simulink model "sampleModel1702_4_sub_sub_sub"  (R2023a)
settings: Solver=VariableStepAuto  StartTime=0.0  StopTime=10.0  RelTol=1e-3
libraries: hdlsllib x4, simulink x2
settings Model: Creator=user1  LastModifiedBy=user1
settings OptimizationCC: BlockReduction=off  ConditionallyExecuteInputs=off

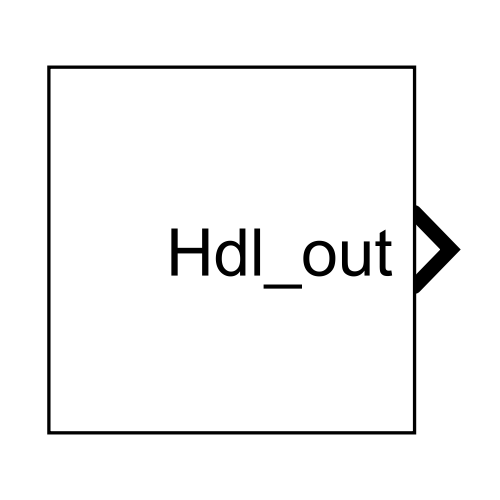
[thumbnail: Simulink's stored preview of the top-level diagram]
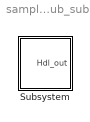
== system sampleModel1702_4_sub_sub_sub ==
  Subsystem : Subsystem

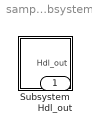
== system sampleModel1702_4_sub_sub_sub/Subsystem ==
  Subsystem : Subsystem
  Hdl_out : Outport  OutDataTypeStr=uint8

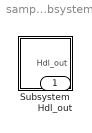
== system sampleModel1702_4_sub_sub_sub/Subsystem/Subsystem ==
  Subsystem : Subsystem
  Hdl_out : Outport  OutDataTypeStr=uint8

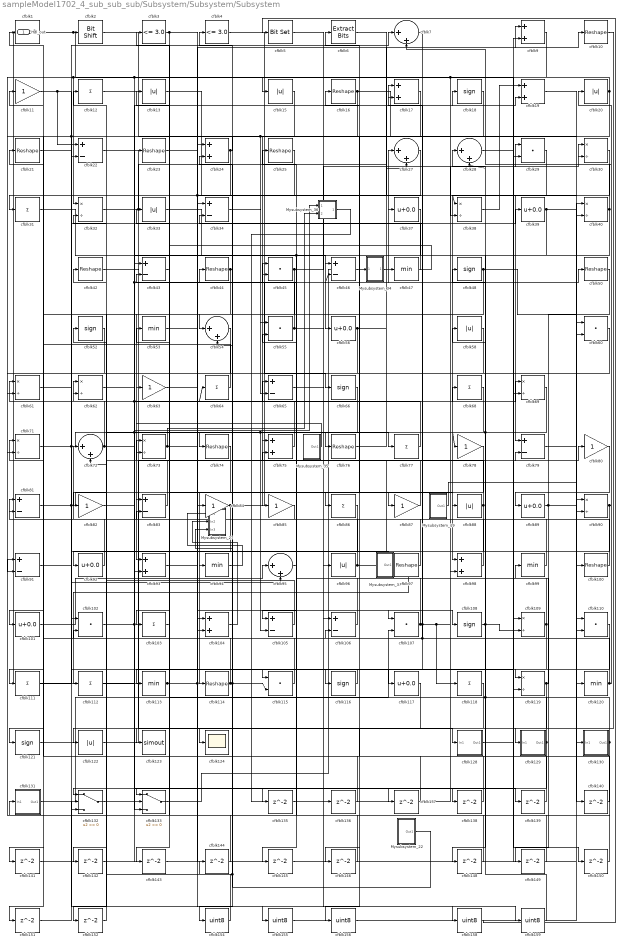
== system sampleModel1702_4_sub_sub_sub/Subsystem/Subsystem/Subsystem ==
  Mysubsystem_19 : Subsystem  TreatAsAtomicUnit=on  RTWFcnName=Mysubsystem_19
      settings: RTWFcnNameOpts=User specified  RTWFileNameOpts=Use function name
  Mysubsystem_22 : Subsystem  TreatAsAtomicUnit=on  RTWFcnName=Mysubsystem_22
      settings: RTWFcnNameOpts=User specified  RTWFileNameOpts=Use function name
  Mysubsystem_27 : Subsystem  TreatAsAtomicUnit=on  RTWFcnName=Mysubsystem_27
      settings: RTWFcnNameOpts=User specified  RTWFileNameOpts=Use function name
  Mysubsystem_34 : Subsystem  TreatAsAtomicUnit=on  RTWFcnName=Mysubsystem_34
      settings: RTWFcnNameOpts=User specified  RTWFileNameOpts=Use function name
  Mysubsystem_35 : Subsystem  TreatAsAtomicUnit=on  RTWFcnName=Mysubsystem_35
      settings: RTWFcnNameOpts=User specified  RTWFileNameOpts=Use function name
  Mysubsystem_36 : Subsystem  TreatAsAtomicUnit=on  RTWFcnName=Mysubsystem_36
      settings: RTWFcnNameOpts=User specified  RTWFileNameOpts=Use function name
  Mysubsystem_37 : Subsystem  TreatAsAtomicUnit=on  RTWFcnName=Mysubsystem_37
      settings: RTWFcnNameOpts=User specified  RTWFileNameOpts=Use function name
  cfblk1 : ArithShift  BitShiftNumber=8
  cfblk{10,16,21,23,25,42,44,50,74,76,97,100,114} (13 alike) : Reshape
  cfblk{37,39,56,89,92,101,117} (7 alike) : Bias  Bias=0.0  SaturateOnIntegerOverflow=off
  cfblk{29,45,55,60,102,107,110,115} (8 alike) : DotProduct  OutDataTypeStr=uint8
  cfblk{12,31,64,68,77,86,103,111..112,118} (10 alike) : Sum  Inputs=+  OutDataTypeStr=uint8
  cfblk{9,17,19,24,75,93,98,104} (8 alike) : Sum  OutDataTypeStr=uint8
  cfblk{22,34,43,46,65,79,81,83,91,105..106} (11 alike) : Sum  Inputs=+-  OutDataTypeStr=uint8
  cfblk{18,48,52,66,108,116,121} (7 alike) : Signum
  cfblk{30,32,38,40,61..62,69,71,73,90,109,119} (12 alike) : Product  Inputs=*/  OutDataTypeStr=uint8  RndMeth=Zero  SaturateOnIntegerOverflow=on
  cfblk{11,63,78,80,82,84..85,87} (8 alike) : Gain  OutDataTypeStr=uint8
  cfblk{47,53,94,99,113,120} (6 alike) : MinMax  OutDataTypeStr=uint8
  cfblk{13,15,20,33,58,88,96,122} (8 alike) : Abs  OutDataTypeStr=uint8  SaturateOnIntegerOverflow=off
  cfblk123 : ToWorkspace  VariableName=simout  SaveFormat=Timeseries  SampleTime=-1
  cfblk124 : Scope
  cfblk128 : Subsystem
      settings: LibrarySourceBlock=|
      | hdlsllib/Ports &
      | Subsystems/Subsystem
  cfblk129 : Subsystem
      settings: LibrarySourceBlock=|
      | hdlsllib/Ports &
      | Subsystems/Subsystem
  cfblk130 : Subsystem
      settings: LibrarySourceBlock=|
      | hdlsllib/Ports &
      | Subsystems/Subsystem
  cfblk131 : Subsystem
      settings: LibrarySourceBlock=|
      | hdlsllib/Ports &
      | Subsystems/Subsystem
  cfblk132 : Switch  OutDataTypeStr=uint8  SaturateOnIntegerOverflow=off  InputSameDT=off
  cfblk133 : Switch  OutDataTypeStr=uint8  SaturateOnIntegerOverflow=off  InputSameDT=off
  cfblk{135..146,148..152} (17 alike) : Delay  SampleTime=1
  cfblk{154..156,158..159} (5 alike) : DataTypeConversion  OutDataTypeStr=uint8  SaturateOnIntegerOverflow=off  RndMeth=Floor
  cfblk2 : hdlsllib/Logic and Bit Operations/Bit Shift  mode=Shift Left Logical  N=0
  cfblk{7,27..28,54,72,95} (6 alike) : Sum  Inputs=|++  OutDataTypeStr=uint8
  cfblk3 : hdlsllib/Logic and Bit Operations/Compare To Constant  relop=<=  const=3.0  OutDataTypeStr=uint8
  cfblk4 : hdlsllib/Logic and Bit Operations/Compare To Constant  relop=<=  const=3.0  OutDataTypeStr=uint8
  cfblk5 : simulink/Logic and Bit Operations/Bit Set  iBit=0
      settings: LibrarySourceBlock=|
      | hdlsllib/Logic and Bit
      | Operations/Bit Set
  cfblk6 : simulink/Logic and Bit Operations/Extract Bits  bitsToExtract=Upper half  numBits=8  bitIdxRange=[0 7]  outScalingMode=Preserve fixed-point scaling
      settings: LibrarySourceBlock=|
      | hdlsllib/Logic and Bit
      | Operations/Extract Bits
  Hdl_out : Outport  OutDataTypeStr=uint8
  wires:
  cfblk122/1 -> cfblk80/1
  cfblk80/1 -> cfblk89/1
  cfblk9/1 -> cfblk38/2, cfblk71/2, cfblk32/1
  cfblk113/1 -> Hdl_out/1, cfblk137/1, cfblk69/1
  cfblk42/1 -> cfblk128/1(In1)
  cfblk72/1 -> cfblk62/1, Mysubsystem_36/1(In1)
  cfblk44/1 -> cfblk54/2, cfblk93/1
  cfblk31/1 -> cfblk56/1
  cfblk88/1 -> cfblk122/1, cfblk16/1
  cfblk105/1 -> cfblk12/1
  cfblk56/1 -> cfblk141/1, cfblk27/2
  cfblk120/1 -> cfblk20/1, cfblk17/1, cfblk71/1
  cfblk10/1 -> cfblk129/1(In1)
  cfblk84/1 -> cfblk104/2, cfblk50/1
  cfblk66/1 -> cfblk74/1
  cfblk71/1 -> cfblk119/2, cfblk77/1
  cfblk22/1 -> cfblk114/1
  cfblk27/1 -> cfblk85/1
  cfblk38/1 -> cfblk19/1
  cfblk30/1 -> cfblk98/1
  cfblk17/1 -> cfblk75/1
  cfblk18/1 -> cfblk86/1
  cfblk81/1 -> cfblk39/1, cfblk88/1
  cfblk74/1 -> cfblk103/1
  cfblk132/1 -> cfblk23/1
  cfblk46/1 -> cfblk27/1
  cfblk25/1 -> cfblk31/1
  cfblk13/1 -> cfblk100/1
  cfblk77/1 -> cfblk61/1
  cfblk48/1 -> cfblk151/1, cfblk60/2
  cfblk4/1 -> cfblk66/1
  cfblk24/1 -> cfblk4/1, cfblk101/1
  cfblk83/1 -> cfblk62/2
  cfblk60/1 -> cfblk92/1
  cfblk39/1 -> cfblk133/3, cfblk130/1(In1)
  cfblk52/1 -> cfblk121/1
  cfblk90/1 -> cfblk105/1, cfblk30/1
  cfblk76/1 -> cfblk19/2
  cfblk85/1 -> cfblk83/2
  cfblk54/1 -> cfblk61/2
  cfblk95/1 -> cfblk45/1
  cfblk16/1 -> cfblk91/2, cfblk90/1
  cfblk115/1 -> cfblk73/1
  cfblk101/1 -> cfblk95/1
  cfblk102/1 -> cfblk139/1, cfblk17/2, cfblk64/1
  cfblk106/1 -> cfblk44/1
  cfblk15/1 -> cfblk124/1
  cfblk33/1 -> cfblk46/1
  cfblk111/1 -> cfblk7/1
  cfblk20/1 -> cfblk15/1, cfblk65/2, cfblk111/1, cfblk22/2
  cfblk103/1 -> cfblk53/1
  cfblk23/1 -> cfblk9/1
  cfblk91/1 -> cfblk102/1
  cfblk43/1 -> cfblk63/1
  cfblk78/1 -> cfblk94/1
  cfblk87/1 -> cfblk73/2
  cfblk3/1 -> cfblk133/1, cfblk155/1, cfblk38/1
  cfblk92/1 -> cfblk81/1
  cfblk2/1 -> cfblk96/1
  cfblk29/1 -> cfblk79/1
  cfblk12/1 -> cfblk109/1
  cfblk93/1 -> cfblk68/1
  cfblk45/1 -> cfblk82/1, cfblk30/2
  cfblk108/1 -> cfblk28/2, cfblk109/2
  cfblk32/1 -> cfblk104/1, cfblk10/1
  cfblk65/1 -> cfblk107/1
  cfblk63/1 -> cfblk47/1
  cfblk99/1 -> cfblk11/1
  cfblk1/1 -> cfblk2/1, cfblk69/2, cfblk43/1
  cfblk40/1 -> cfblk7/2, cfblk148/1, cfblk78/1
  cfblk64/1 -> cfblk21/1
  cfblk34/1 -> cfblk55/1
  cfblk96/1 -> cfblk79/2, cfblk42/1
  cfblk121/1 -> cfblk107/2
  cfblk37/1 -> cfblk145/1, cfblk54/1
  cfblk61/1 -> cfblk97/1
  cfblk11/1 -> cfblk22/1, cfblk95/2
  cfblk116/1 -> cfblk113/1
  cfblk98/1 -> cfblk72/1
  cfblk19/1 -> cfblk90/2
  cfblk86/1 -> cfblk115/1
  cfblk112/1 -> cfblk46/2, cfblk18/1
  cfblk55/1 -> cfblk13/1, cfblk106/1
  cfblk47/1 -> cfblk34/2
  cfblk89/1 -> cfblk149/1, cfblk40/1
  cfblk100/1 -> cfblk28/1
  cfblk131/1(Out1) -> cfblk84/1
  cfblk82/1 -> cfblk116/1
  cfblk53/1 -> cfblk108/1
  cfblk7/1 -> cfblk117/1
  cfblk68/1 -> cfblk105/2, cfblk133/2, cfblk132/1
  cfblk58/1 -> cfblk87/1
  cfblk130/1(Out1) -> cfblk6/1, cfblk131/1(In1)
  cfblk75/1 -> cfblk65/1
  cfblk119/1 -> cfblk156/1, cfblk99/1
  cfblk109/1 -> cfblk45/2, cfblk123/1
  cfblk97/1 -> cfblk3/1
  cfblk114/1 -> cfblk52/1, cfblk24/2, cfblk115/2
  cfblk107/1 -> cfblk25/1, cfblk37/1, cfblk118/1, cfblk29/1
  cfblk129/1(Out1) -> cfblk152/1, cfblk33/1, cfblk48/1
  cfblk128/1(Out1) -> cfblk29/2
  cfblk6/1 -> cfblk40/2
  cfblk73/1 -> cfblk76/1, Mysubsystem_36/2(In2)
  cfblk50/1 -> cfblk119/1
  cfblk62/1 -> cfblk135/1
  cfblk135/1 -> cfblk98/2
  cfblk136/1 -> cfblk72/2
  cfblk137/1 -> cfblk1/1
  cfblk69/1 -> cfblk138/1
  cfblk138/1 -> cfblk81/2
  cfblk139/1 -> cfblk106/2
  cfblk79/1 -> cfblk140/1
  cfblk140/1 -> cfblk75/2
  cfblk141/1 -> cfblk60/1
  cfblk118/1 -> cfblk142/1
  cfblk142/1 -> cfblk93/2
  cfblk143/1 -> cfblk34/1
  cfblk144/1 -> cfblk91/1
  cfblk145/1 -> cfblk9/2
  cfblk117/1 -> cfblk146/1
  cfblk146/1 -> cfblk55/2
  cfblk148/1 -> cfblk43/2
  cfblk149/1 -> cfblk132/2
  cfblk28/1 -> cfblk150/1
  cfblk150/1 -> cfblk24/1
  cfblk151/1 -> cfblk132/3
  cfblk152/1 -> cfblk32/2
  cfblk110/1 -> cfblk154/1
  cfblk154/1 -> cfblk144/1
  cfblk155/1 -> cfblk110/1
  cfblk156/1 -> cfblk110/2
  cfblk21/1 -> cfblk158/1
  cfblk158/1 -> cfblk5/1
  cfblk5/1 -> cfblk159/1
  cfblk159/1 -> cfblk58/1
  Mysubsystem_19/1(Out1) -> cfblk120/1
  Mysubsystem_22/1(Out1) -> cfblk102/2, Mysubsystem_27/3(In3)
  cfblk94/1 -> Mysubsystem_27/1(In1)
  cfblk104/1 -> Mysubsystem_27/2(In2)
  cfblk133/1 -> Mysubsystem_34/1(In1)
  Mysubsystem_34/1(Out1) -> cfblk143/1
  Mysubsystem_35/1(Out1) -> cfblk83/1
  Mysubsystem_36/1(Out1) -> cfblk136/1
  Mysubsystem_37/1(Out1) -> cfblk112/1

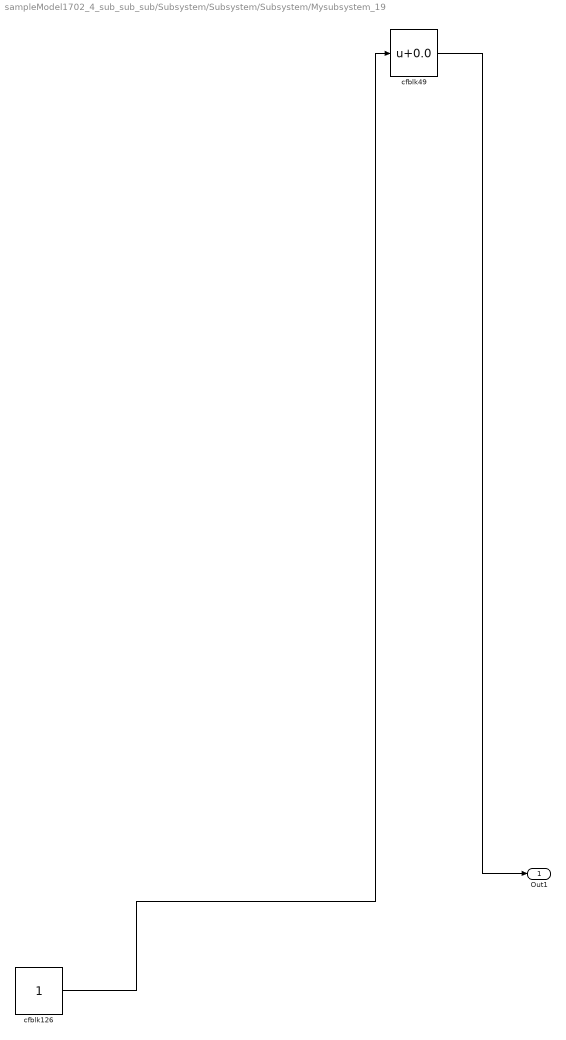
== system sampleModel1702_4_sub_sub_sub/Subsystem/Subsystem/Subsystem/Mysubsystem_19 ==
  cfblk126 : Constant  SampleTime=-1
  cfblk49 : Bias  Bias=0.0  SaturateOnIntegerOverflow=off
  Out1 : Outport
  wires:
  cfblk49/1 -> Out1/1
  cfblk126/1 -> cfblk49/1

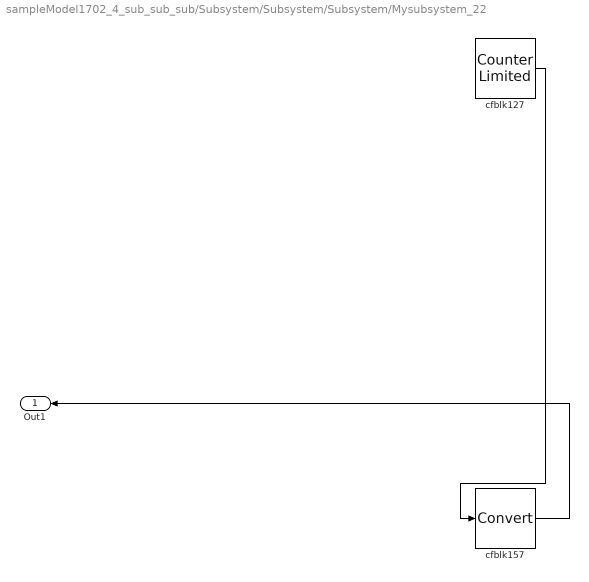
== system sampleModel1702_4_sub_sub_sub/Subsystem/Subsystem/Subsystem/Mysubsystem_22 ==
  cfblk127 : hdlsllib/Sources/Counter Limited  uplimit=7  tsamp=-1
  cfblk157 : DataTypeConversion  SaturateOnIntegerOverflow=off  RndMeth=Floor
  Out1 : Outport
  wires:
  cfblk157/1 -> Out1/1
  cfblk127/1 -> cfblk157/1

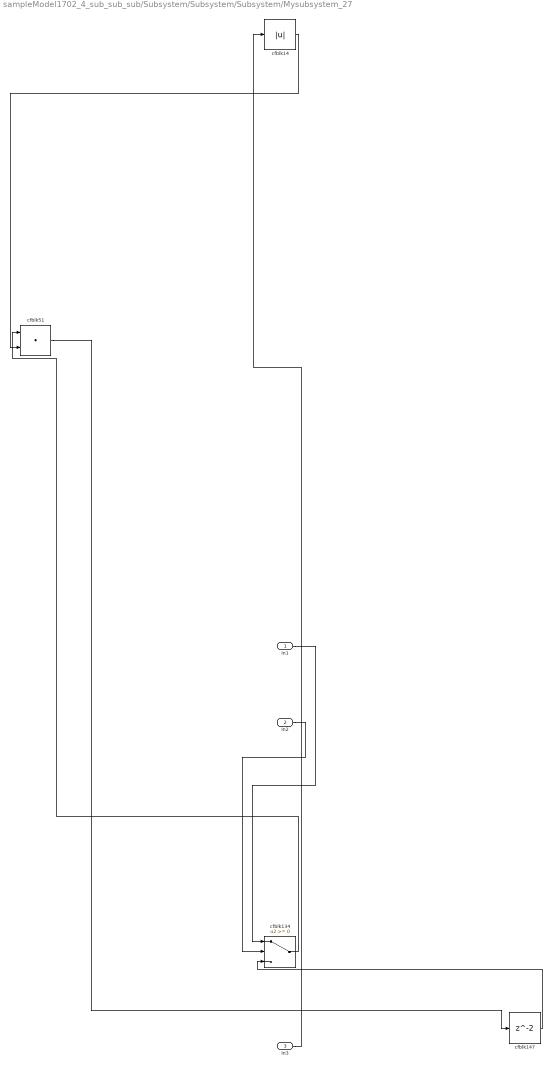
== system sampleModel1702_4_sub_sub_sub/Subsystem/Subsystem/Subsystem/Mysubsystem_27 ==
  In1 : Inport
  In2 : Inport  Port=2
  In3 : Inport  Port=3
  cfblk134 : Switch  SaturateOnIntegerOverflow=off  InputSameDT=off
  cfblk14 : Abs  SaturateOnIntegerOverflow=off
  cfblk147 : Delay  SampleTime=1
  cfblk51 : DotProduct  OutDataTypeStr=Inherit: Inherit via internal rule
  wires:
  In3/1 -> cfblk14/1
  cfblk134/1 -> cfblk51/1
  cfblk147/1 -> cfblk134/3
  In2/1 -> cfblk134/2
  cfblk51/1 -> cfblk147/1
  cfblk14/1 -> cfblk51/2
  In1/1 -> cfblk134/1

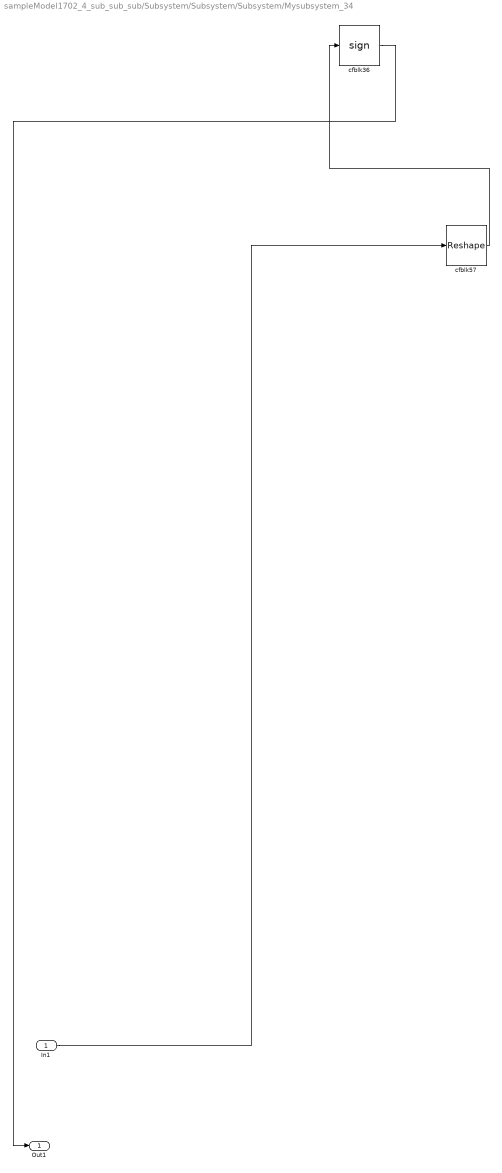
== system sampleModel1702_4_sub_sub_sub/Subsystem/Subsystem/Subsystem/Mysubsystem_34 ==
  In1 : Inport
  cfblk36 : Signum
  cfblk57 : Reshape
  Out1 : Outport
  wires:
  cfblk36/1 -> Out1/1
  In1/1 -> cfblk57/1
  cfblk57/1 -> cfblk36/1

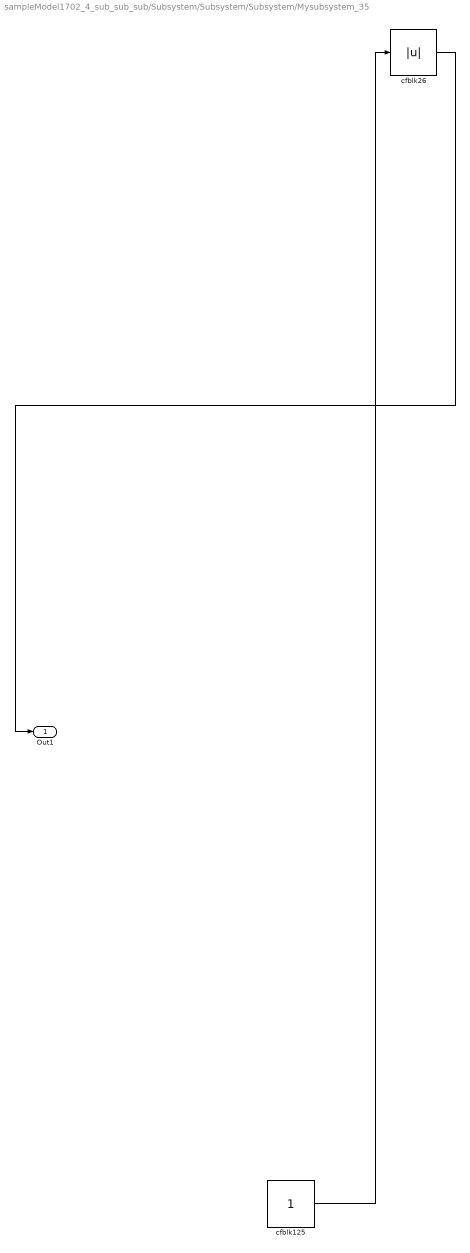
== system sampleModel1702_4_sub_sub_sub/Subsystem/Subsystem/Subsystem/Mysubsystem_35 ==
  cfblk125 : Constant  SampleTime=-1
  cfblk26 : Abs  SaturateOnIntegerOverflow=off
  Out1 : Outport
  wires:
  cfblk26/1 -> Out1/1
  cfblk125/1 -> cfblk26/1

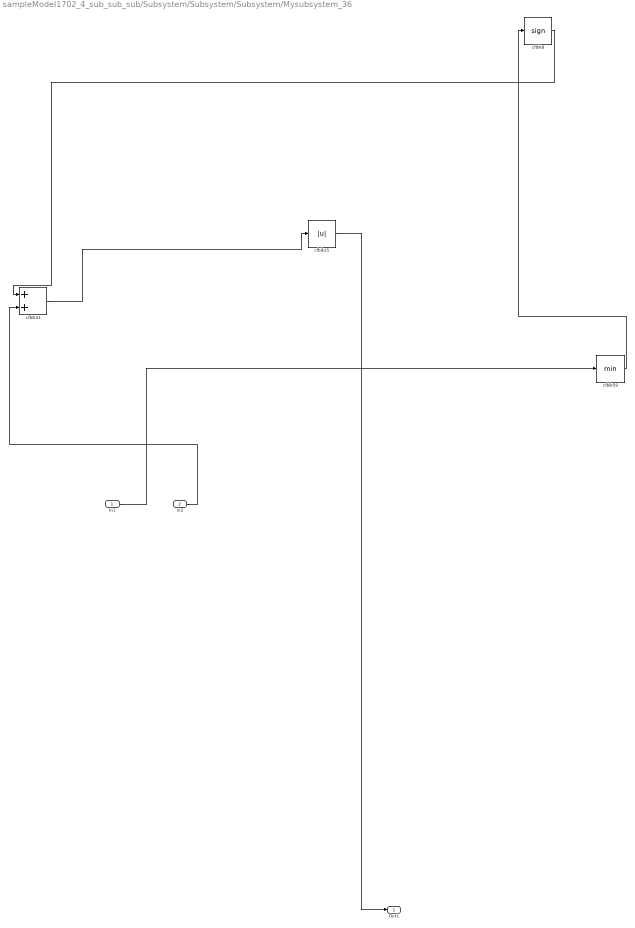
== system sampleModel1702_4_sub_sub_sub/Subsystem/Subsystem/Subsystem/Mysubsystem_36 ==
  In1 : Inport
  In2 : Inport  Port=2
  cfblk35 : Abs  SaturateOnIntegerOverflow=off
  cfblk41 : Sum
  cfblk59 : MinMax
  cfblk8 : Signum
  Out1 : Outport
  wires:
  cfblk59/1 -> cfblk8/1
  cfblk35/1 -> Out1/1
  cfblk41/1 -> cfblk35/1
  In1/1 -> cfblk59/1
  In2/1 -> cfblk41/2
  cfblk8/1 -> cfblk41/1

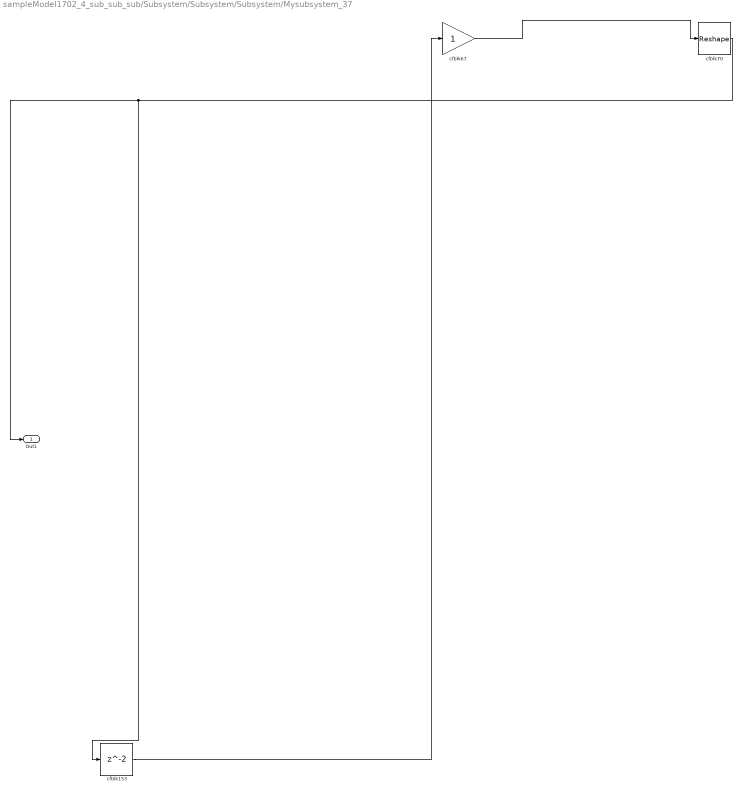
== system sampleModel1702_4_sub_sub_sub/Subsystem/Subsystem/Subsystem/Mysubsystem_37 ==
  cfblk153 : Delay  SampleTime=1
  cfblk67 : Gain
  cfblk70 : Reshape
  Out1 : Outport
  wires:
  cfblk153/1 -> cfblk67/1
  cfblk67/1 -> cfblk70/1
  cfblk70/1 -> cfblk153/1, Out1/1

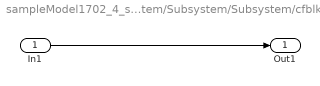
== system sampleModel1702_4_sub_sub_sub/Subsystem/Subsystem/Subsystem/cfblk128 ==
  In1 : Inport
  Out1 : Outport
  wires:
  In1/1 -> Out1/1

== system sampleModel1702_4_sub_sub_sub/Subsystem/Subsystem/Subsystem/cfblk129 ==
  In1 : Inport
  Out1 : Outport
  wires:
  In1/1 -> Out1/1

== system sampleModel1702_4_sub_sub_sub/Subsystem/Subsystem/Subsystem/cfblk130 ==
  In1 : Inport
  Out1 : Outport
  wires:
  In1/1 -> Out1/1

== system sampleModel1702_4_sub_sub_sub/Subsystem/Subsystem/Subsystem/cfblk131 ==
  In1 : Inport
  Out1 : Outport
  wires:
  In1/1 -> Out1/1
